simulink model "SPWM"  (R2019b)
settings: Solver=ode1  StartTime=0.0  StopTime=2  FixedStep=1e-5  RelTol=1e-3
InitFcn:
  | %T=0.0000071
  | T = (1e-5)/2
  | 
  | flux=0.2068
values from neighbouring files (symbols this model uses):
  B = 0.0136    [Pmsm.m]
  J = 0.0027    [Pmsm.m]
  Kiq = double(Kiq)    [Pmsm.m]
  Kiw = double(Kiw)    [Pmsm.m]
  Kpq = double(Kpq)    [Pmsm.m]
  Kpw = double(Kpw)    [Pmsm.m]
  Lambda_m = 0.2026    [Pmsm.m]
  Ld = 19.75e-3    (= 0.01975)    [Pmsm.m]
  Lq = 22.5e-3    (= 0.0225)    [Pmsm.m]
  P = 8    [Pmsm.m]
  Rs = 1.477    [Pmsm.m]
  Vdc = 220    [Pmsm.m]
libraries: modelsimlib x1
settings Model: Creator=samfi  LastModifiedBy=samfi

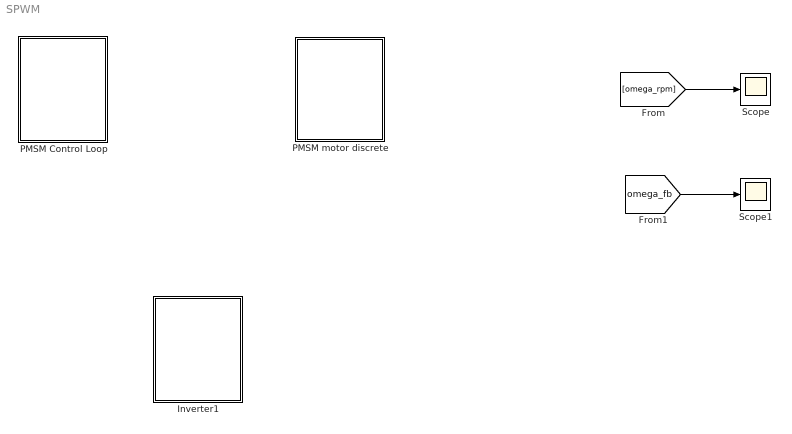
== system SPWM ==
  Inverter1 : Subsystem
  PMSM Control Loop : Subsystem
  PMSM motor discrete : Subsystem
  Scope : Scope
  Scope1 : Scope
  wires:
  [omega_rpm] -> Scope/1
  [omega_fb] -> Scope1/1

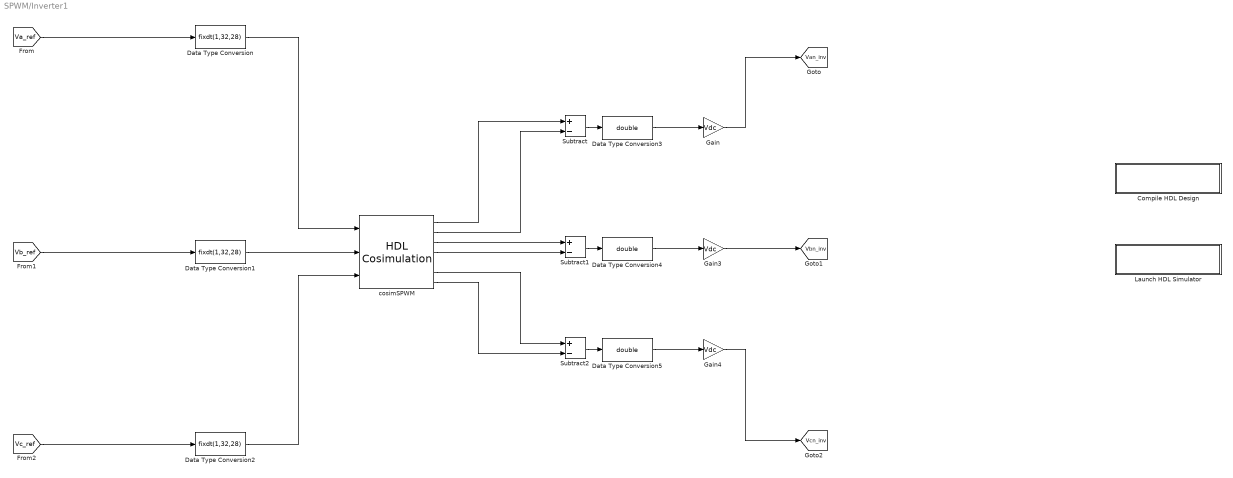
== system SPWM/Inverter1 ==
  Compile HDL Design : Subsystem
      settings: OpenFcn=eval('compile_hdl_design_cosimSPWM');
      mask Display: disp(['Double-Click to' char(10) 'compile HDL files'])
  Data Type Conversion : DataTypeConversion  OutDataTypeStr=fixdt(1,32,28)
  Data Type Conversion1 : DataTypeConversion  OutDataTypeStr=fixdt(1,32,28)
  Data Type Conversion2 : DataTypeConversion  OutDataTypeStr=fixdt(1,32,28)
  Data Type Conversion3 : DataTypeConversion  OutDataTypeStr=double
  Data Type Conversion4 : DataTypeConversion  OutDataTypeStr=double
  Data Type Conversion5 : DataTypeConversion  OutDataTypeStr=double
  Gain : Gain  Gain=Vdc
  Gain3 : Gain  Gain=Vdc
  Gain4 : Gain  Gain=Vdc
  Launch HDL Simulator : Subsystem
      settings: OpenFcn=eval('launch_hdl_simulator_cosimSPWM');
      mask Display: disp(['Double-Click to' char(10) 'launch HDL simulator'])
  Subtract : Sum  Inputs=+-
  Subtract1 : Sum  Inputs=+-
  Subtract2 : Sum  Inputs=+-
  cosimSPWM : modelsimlib/HDL Cosimulation  PortPaths=/cosimSPWM/x;/cosimSPWM/y;/cosimSPWM/z;/cosimSPWM/Sau;/cosimSPWM/Sal;/cosimSPWM/Sbu;/cosimSPWM/Sbl;/cosimSPWM/Scu;/cosimSPWM/Scl;/cosimSPWM/out;  PortModes=[1 1 1 2 2 2 2 2 2 2 ]  PortTimes=[-1,-1,-1,1e-4,1e-4,1e-4,1e-4,1e-4,1e-4,1e-4]  PortSigns=[-1,-1,-1,-1,-1,-1,-1,-1,-1,-1,]  PortFracLengths=[0,0,0,0,0,0,0,0,0,0]  CommLocal=on  CommSharedMemory=on  CommPortNumber=4449  CommShowInfo=on  ClockModes=[]  ClockTimes=[]  TclPreSimCommand=|  TclPostSimCommand=|  TimingMode=s  TimingScaleFactor=1  idxCellArray={'UNUSED_VAR'}  CosimBypass=Full Simulation  AllowDirectFeedthrough=on  ProductName=EDA Simulator Link MQ  RunAutoTimescale=on  HdlClocks=/cosimSPWM/clk 10 ns;  PreRunTime=10  PreRunTimeUnit=ns
      TclPreSimCommand=|
      | force /cosimSPWM/clk 0 0 ns, 1 5 ns -repeat 10 ns;
      | force /cosimSPWM/res 1 0 ns, 0 8 ns;
      TclPostSimCommand=|
      | noforce /cosimSPWM/clk;
      | noforce /cosimSPWM/res;
      | puts "done";
      settings: SourceProductName=HDL Verifier  SourceProductBaseCode=ES
  tag scope: Van_inv=global, Vbn_inv=global, Vcn_inv=global
  wires:
  [Vc_ref] -> Data Type Conversion2/1
  [Vb_ref] -> Data Type Conversion1/1
  [Va_ref] -> Data Type Conversion/1
  Data Type Conversion/1 -> cosimSPWM/1
  Data Type Conversion1/1 -> cosimSPWM/2
  Data Type Conversion2/1 -> cosimSPWM/3
  cosimSPWM/1 -> Subtract/1
  cosimSPWM/2 -> Subtract/2
  cosimSPWM/3 -> Subtract1/1
  cosimSPWM/4 -> Subtract1/2
  cosimSPWM/6 -> Subtract2/1
  cosimSPWM/7 -> Subtract2/2
  Subtract/1 -> Data Type Conversion3/1
  Subtract1/1 -> Data Type Conversion4/1
  Subtract2/1 -> Data Type Conversion5/1
  Gain4/1 -> [Vcn_inv]
  Gain3/1 -> [Vbn_inv]
  Gain/1 -> [Van_inv]
  Data Type Conversion3/1 -> Gain/1
  Data Type Conversion4/1 -> Gain3/1
  Data Type Conversion5/1 -> Gain4/1

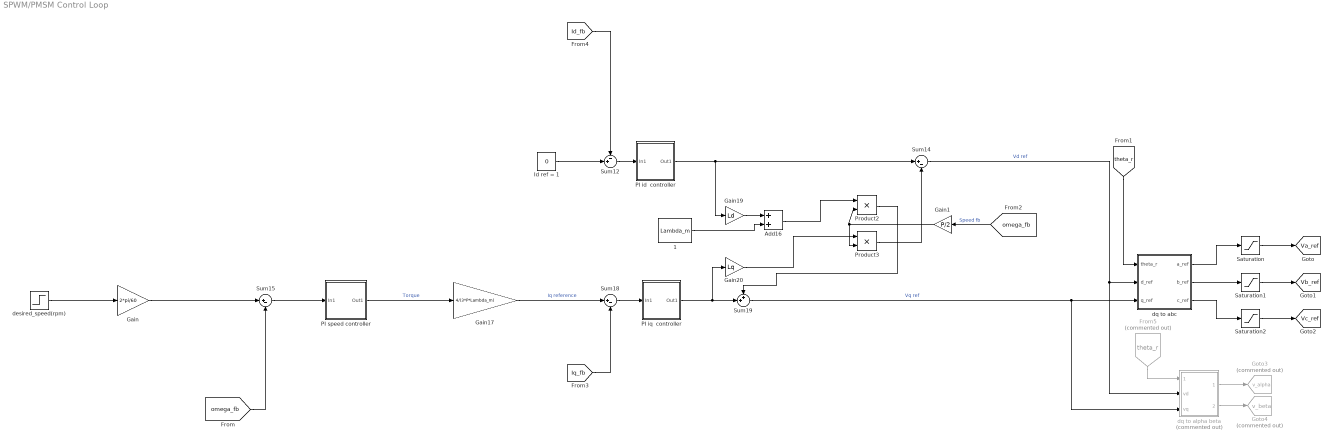
== system SPWM/PMSM Control Loop ==
  " 1" : Constant  Value=Lambda_m  SampleTime=1e-4
  Add16 : Sum
  From5 : From  Commented=on  GotoTag=theta_r  TagVisibility=global
  Gain : Gain  Gain=2*pi/60
  Gain1 : Gain  Gain=P/2
  Gain17 : Gain  Gain=4/(3*P*Lambda_m)
  Gain19 : Gain  Gain=Ld
  Gain20 : Gain  Gain=Lq
  Goto3 : Goto  Commented=on  GotoTag=v_alpha  TagVisibility=global
  Goto4 : Goto  Commented=on  GotoTag=v_beta  TagVisibility=global
  Id ref = 1 : Constant  Value=0  SampleTime=1e-4
  PI id  controller : Subsystem
  PI iq  controller : Subsystem
  PI speed controller : Subsystem
  Product2 : Product
  Product3 : Product
  Saturation : Saturate  UpperLimit=200  LowerLimit=-200
  Saturation1 : Saturate  UpperLimit=200  LowerLimit=-200
  Saturation2 : Saturate  UpperLimit=200  LowerLimit=-200
  Sum12 : Sum  Inputs=-+|
  Sum14 : Sum  Inputs=|+-
  Sum15 : Sum  Inputs=|+-
  Sum18 : Sum  Inputs=|+-
  Sum19 : Sum  Inputs=++|
  desired_speed(rpm) : Step  Time=0.25  After=400  SampleTime=1e-4
  dq to abc : Subsystem
  dq to alpha beta : Subsystem  Commented=on
  tag scope: Va_ref=global, Vb_ref=global, Vc_ref=global
  wires:
  Product2/1 -> Sum19/1
  Add16/1 -> Product2/1
  Gain20/1 -> Product3/1
  Product3/1 -> Sum14/2
  Id ref = 1/1 -> Sum12/2
  PI iq  controller/1(Out1) -> Gain20/1, Sum19/2
  PI id  controller/1(Out1) -> Gain19/1, Sum14/1
  Sum14/1 -> dq to alpha beta/2(vd), dq to abc/2(d_ref)  "Vd ref"
  Gain19/1 -> Add16/1
  Sum18/1 -> PI iq  controller/1(In1)
  " 1"/1 -> Add16/2
  Gain17/1 -> Sum18/1  "Iq reference"
  Sum19/1 -> dq to alpha beta/3(vq), dq to abc/3(q_ref)  "Vq ref"
  [omega_fb] -> Sum15/2
  [theta_r] -> dq to abc/1(theta_r)
  [Iq_fb] -> Sum18/2
  [Id_fb] -> Sum12/1
  Saturation/1 -> [Va_ref]
  Saturation1/1 -> [Vb_ref]
  Saturation2/1 -> [Vc_ref]
  dq to abc/3(c_ref) -> Saturation2/1
  dq to abc/1(a_ref) -> Saturation/1
  dq to abc/2(b_ref) -> Saturation1/1
  Gain/1 -> Sum15/1
  [omega_fb] -> Gain1/1  "Speed fb"
  Gain1/1 -> Product3/2, Product2/2
  Sum12/1 -> PI id  controller/1(In1)
  Sum15/1 -> PI speed controller/1(In1)
  PI speed controller/1(Out1) -> Gain17/1  "Torque"
  dq to alpha beta/1(valpha) -> Goto3/1
  dq to alpha beta/2(vbeta) -> Goto4/1
  From5/1 -> dq to alpha beta/1(theta_r)
  desired_speed(rpm)/1 -> Gain/1

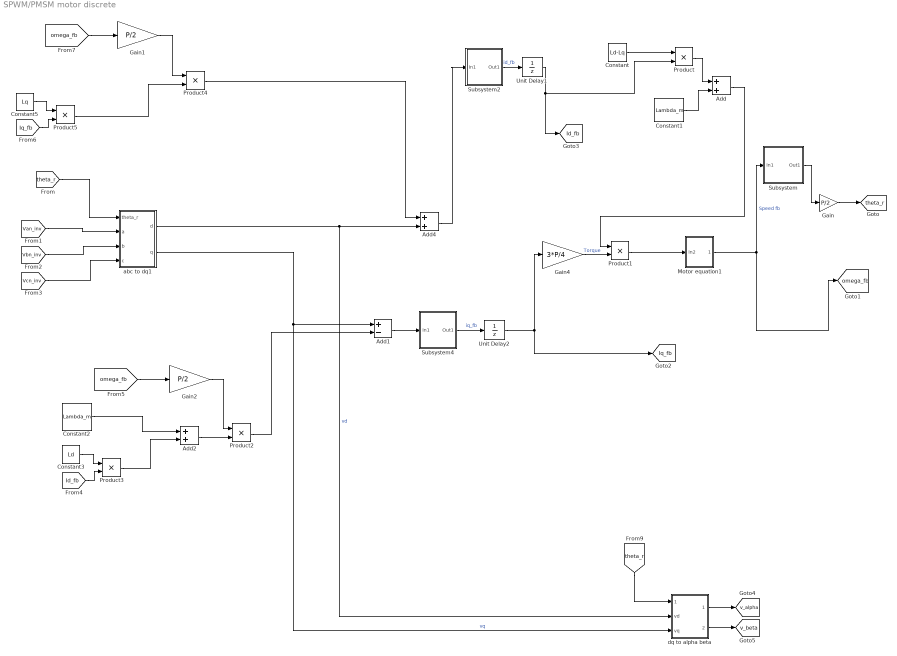
== system SPWM/PMSM motor discrete ==
  Add : Sum
  Add1 : Sum  Inputs=+-
  Add2 : Sum
  Add4 : Sum
  Constant : Constant  Value=Ld-Lq  SampleTime=1e-4
  Constant1 : Constant  Value=Lambda_m  SampleTime=1e-4
  Constant2 : Constant  Value=Lambda_m  SampleTime=1e-4
  Constant3 : Constant  Value=Ld  SampleTime=1e-4
  Constant5 : Constant  Value=Lq  SampleTime=1e-4
  Gain : Gain  Gain=P/2
  Gain1 : Gain  Gain=P/2
  Gain2 : Gain  Gain=P/2
  Gain4 : Gain  Gain=3*P/4
  Motor equation1 : Subsystem
  Product{,1..5} (6 alike) : Product
  Subsystem : Subsystem
  Subsystem2 : Subsystem
  Subsystem4 : Subsystem
  Unit Delay1 : UnitDelay  SampleTime=-1  HasFrameUpgradeWarning=on
  Unit Delay2 : UnitDelay  SampleTime=-1  HasFrameUpgradeWarning=on
  abc to dq1 : Subsystem
  dq to alpha beta : Subsystem
  tag scope: Id_fb=global, Iq_fb=global, omega_fb=global, theta_r=global, v_alpha=global, v_beta=global
  wires:
  Subsystem4/1(Out1) -> Unit Delay2/1  "iq_fb"
  [Vbn_inv] -> abc to dq1/3(b)
  Motor equation1/1(Out1) -> [omega_fb], Subsystem/1(In1)  "Speed fb"
  [Van_inv] -> abc to dq1/2(a)
  [Vcn_inv] -> abc to dq1/4(c)
  Subsystem2/1(Out1) -> Unit Delay1/1  "id_fb"
  Product1/1 -> Motor equation1/1(In2)
  Constant/1 -> Product/1
  Product/1 -> Add/1
  Constant1/1 -> Add/2
  Gain4/1 -> Product1/2  "Torque"
  Add/1 -> Product1/1
  Subsystem/1(Out1) -> Gain/1
  Gain/1 -> [theta_r]
  abc to dq1/2(q) -> dq to alpha beta/3(vq), Add1/1  "vq"
  Product2/1 -> Add1/2
  [omega_fb] -> Gain2/1
  Constant3/1 -> Product3/1
  [Id_fb] -> Product3/2
  Product3/1 -> Add2/2
  Constant2/1 -> Add2/1
  Add2/1 -> Product2/2
  [Iq_fb] -> Product5/2
  Product5/1 -> Product4/2
  Constant5/1 -> Product5/1
  abc to dq1/1(d) -> dq to alpha beta/2(vd), Add4/2  "vd"
  Product4/1 -> Add4/1
  [omega_fb] -> Gain1/1
  Gain1/1 -> Product4/1
  Gain2/1 -> Product2/1
  dq to alpha beta/1(valpha) -> [v_alpha]
  dq to alpha beta/2(vbeta) -> [v_beta]
  [theta_r] -> abc to dq1/1(theta_r)
  [theta_r] -> dq to alpha beta/1(theta_r)
  Add4/1 -> Subsystem2/1(In1)
  Add1/1 -> Subsystem4/1(In1)
  Unit Delay1/1 -> [Id_fb], Product/2
  Unit Delay2/1 -> Gain4/1, [Iq_fb]

== system SPWM/Inverter1/Compile HDL Design ==

== system SPWM/Inverter1/Launch HDL Simulator ==

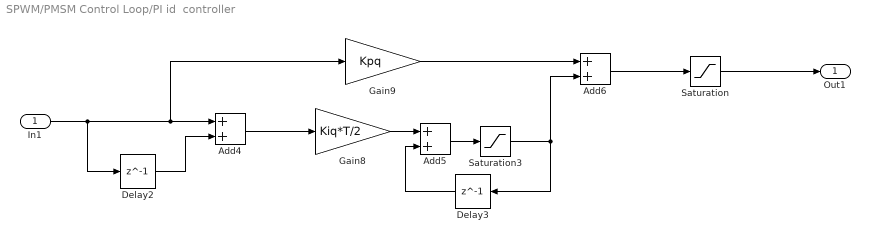
== system SPWM/PMSM Control Loop/PI id  controller ==
  In1 : Inport
  Add4 : Sum
  Add5 : Sum
  Add6 : Sum
  Delay2 : Delay  DelayLength=1
  Delay3 : Delay  DelayLength=1
  Gain8 : Gain  Gain=Kiq*T/2
  Gain9 : Gain  Gain=Kpq
  Saturation : Saturate  UpperLimit=220  LowerLimit=-220
  Saturation3 : Saturate  UpperLimit=200  LowerLimit=-200
  Out1 : Outport
  wires:
  Gain8/1 -> Add5/1
  Delay2/1 -> Add4/2
  Add5/1 -> Saturation3/1
  Add4/1 -> Gain8/1
  Saturation3/1 -> Delay3/1, Add6/2
  In1/1 -> Add4/1, Gain9/1, Delay2/1
  Gain9/1 -> Add6/1
  Delay3/1 -> Add5/2
  Add6/1 -> Saturation/1
  Saturation/1 -> Out1/1

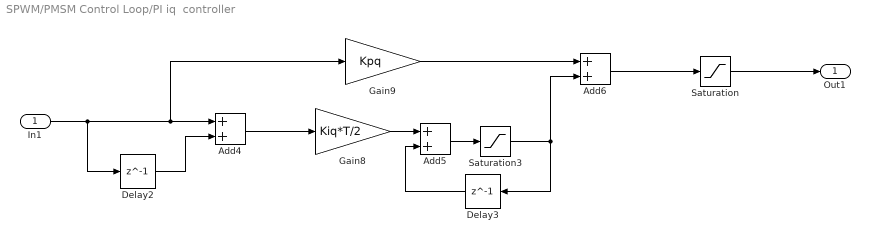
== system SPWM/PMSM Control Loop/PI iq  controller ==
  In1 : Inport
  Add4 : Sum
  Add5 : Sum
  Add6 : Sum
  Delay2 : Delay  DelayLength=1
  Delay3 : Delay  DelayLength=1
  Gain8 : Gain  Gain=Kiq*T/2
  Gain9 : Gain  Gain=Kpq
  Saturation : Saturate  UpperLimit=220  LowerLimit=-220
  Saturation3 : Saturate  UpperLimit=200  LowerLimit=-200
  Out1 : Outport
  wires:
  Delay3/1 -> Add5/2
  Gain9/1 -> Add6/1
  In1/1 -> Delay2/1, Gain9/1, Add4/1
  Saturation3/1 -> Add6/2, Delay3/1
  Add4/1 -> Gain8/1
  Add5/1 -> Saturation3/1
  Delay2/1 -> Add4/2
  Gain8/1 -> Add5/1
  Add6/1 -> Saturation/1
  Saturation/1 -> Out1/1

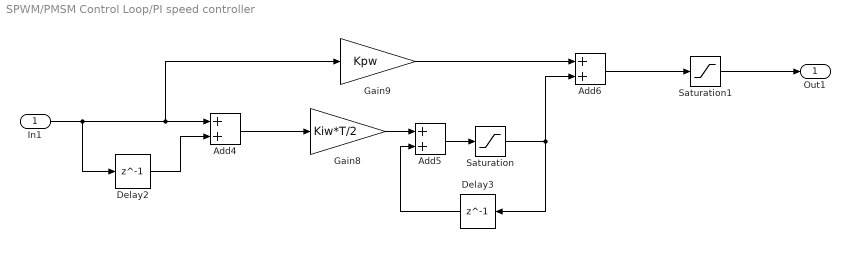
== system SPWM/PMSM Control Loop/PI speed controller ==
  In1 : Inport
  Add4 : Sum
  Add5 : Sum
  Add6 : Sum
  Delay2 : Delay  DelayLength=1
  Delay3 : Delay  DelayLength=1
  Gain8 : Gain  Gain=Kiw*T/2
  Gain9 : Gain  Gain=Kpw
  Saturation : Saturate  UpperLimit=10  LowerLimit=-10
  Saturation1 : Saturate  UpperLimit=10  LowerLimit=-10
  Out1 : Outport
  wires:
  Gain9/1 -> Add6/1
  Delay2/1 -> Add4/2
  Gain8/1 -> Add5/1
  Add5/1 -> Saturation/1
  In1/1 -> Delay2/1, Gain9/1, Add4/1
  Saturation/1 -> Add6/2, Delay3/1
  Add4/1 -> Gain8/1
  Delay3/1 -> Add5/2
  Add6/1 -> Saturation1/1
  Saturation1/1 -> Out1/1

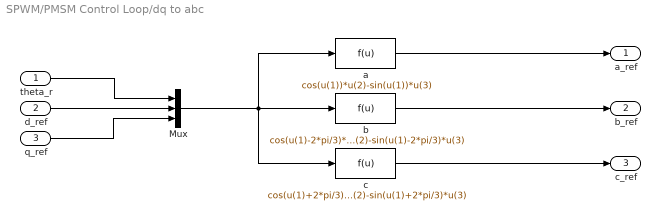
== system SPWM/PMSM Control Loop/dq to abc ==
  theta_r : Inport
  d_ref : Inport  Port=2
  q_ref : Inport  Port=3
  Mux : Mux  Inputs=3
  a : Fcn  Expr=cos(u(1))*u(2)-sin(u(1))*u(3)
  b : Fcn  Expr=cos(u(1)-2*pi/3)*u(2)-sin(u(1)-2*pi/3)*u(3)
  c : Fcn  Expr=cos(u(1)+2*pi/3)*u(2)-sin(u(1)+2*pi/3)*u(3)
  a_ref : Outport
  b_ref : Outport  Port=2
  c_ref : Outport  Port=3
  wires:
  d_ref/1 -> Mux/2
  Mux/1 -> c/1, b/1, a/1
  c/1 -> c_ref/1
  theta_r/1 -> Mux/1
  b/1 -> b_ref/1
  a/1 -> a_ref/1
  q_ref/1 -> Mux/3

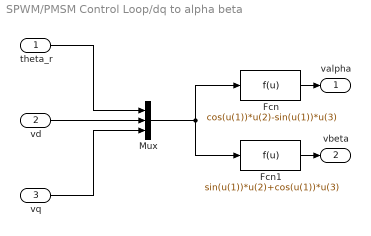
== system SPWM/PMSM Control Loop/dq to alpha beta ==
  theta_r : Inport
  vd : Inport  Port=2
  vq : Inport  Port=3
  Fcn : Fcn  Expr=cos(u(1))*u(2)-sin(u(1))*u(3)
  Fcn1 : Fcn  Expr=sin(u(1))*u(2)+cos(u(1))*u(3)
  Mux : Mux  Inputs=3
  valpha : Outport
  vbeta : Outport  Port=2
  wires:
  Mux/1 -> Fcn/1, Fcn1/1
  vq/1 -> Mux/3
  theta_r/1 -> Mux/1
  Fcn1/1 -> vbeta/1
  vd/1 -> Mux/2
  Fcn/1 -> valpha/1

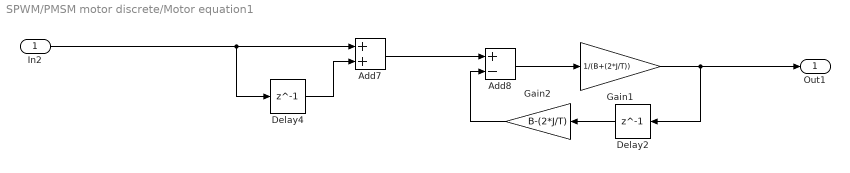
== system SPWM/PMSM motor discrete/Motor equation1 ==
  In2 : Inport
  Add7 : Sum
  Add8 : Sum  Inputs=+-
  Delay2 : Delay  DelayLength=1
  Delay4 : Delay  DelayLength=1
  Gain1 : Gain  Gain=1/(B+(2*J/T))
  Gain2 : Gain  Gain=B-(2*J/T)
  Out1 : Outport
  wires:
  Add7/1 -> Add8/1
  Gain1/1 -> Out1/1, Delay2/1
  Delay2/1 -> Gain2/1
  Add8/1 -> Gain1/1
  Gain2/1 -> Add8/2
  In2/1 -> Delay4/1, Add7/1
  Delay4/1 -> Add7/2

== system SPWM/PMSM motor discrete/Subsystem ==
  In1 : Inport
  Add1 : Sum
  Add2 : Sum
  Delay1 : Delay  DelayLength=1
  Delay4 : Delay  DelayLength=1
  Gain : Gain  Gain=T/2
  Out1 : Outport
  wires:
  In1/1 -> Delay4/1, Add1/1
  Delay1/1 -> Add2/2
  Add2/1 -> Out1/1, Delay1/1
  Delay4/1 -> Add1/2
  Add1/1 -> Gain/1
  Gain/1 -> Add2/1

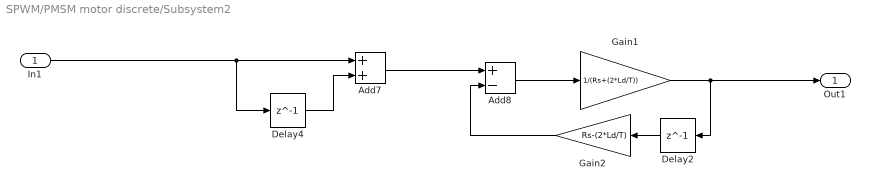
== system SPWM/PMSM motor discrete/Subsystem2 ==
  In1 : Inport
  Add7 : Sum
  Add8 : Sum  Inputs=+-
  Delay2 : Delay  DelayLength=1
  Delay4 : Delay  DelayLength=1
  Gain1 : Gain  Gain=1/(Rs+(2*Ld/T))
  Gain2 : Gain  Gain=Rs-(2*Ld/T)
  Out1 : Outport
  wires:
  Add8/1 -> Gain1/1
  In1/1 -> Add7/1, Delay4/1
  Gain2/1 -> Add8/2
  Delay2/1 -> Gain2/1
  Delay4/1 -> Add7/2
  Add7/1 -> Add8/1
  Gain1/1 -> Out1/1, Delay2/1

== system SPWM/PMSM motor discrete/Subsystem4 ==
  In1 : Inport
  Add7 : Sum
  Add8 : Sum  Inputs=+-
  Delay2 : Delay  DelayLength=1
  Delay4 : Delay  DelayLength=1
  Gain1 : Gain  Gain=1/(Rs+(2*Lq/T))
  Gain2 : Gain  Gain=Rs-(2*Lq/T)
  Out1 : Outport
  wires:
  Add8/1 -> Gain1/1
  Gain1/1 -> Delay2/1, Out1/1
  Add7/1 -> Add8/1
  Delay4/1 -> Add7/2
  Delay2/1 -> Gain2/1
  Gain2/1 -> Add8/2
  In1/1 -> Delay4/1, Add7/1

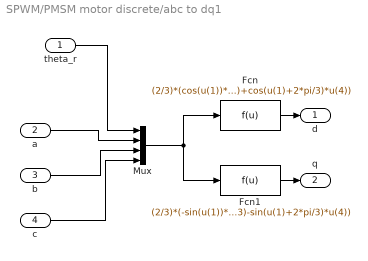
== system SPWM/PMSM motor discrete/abc to dq1 ==
  theta_r : Inport
  a : Inport  Port=2
  b : Inport  Port=3
  c : Inport  Port=4
  Fcn : Fcn  Expr=(2/3)*(cos(u(1))*u(2)+cos(u(1)-2*pi/3)*u(3)+cos(u(1)+2*pi/3)*u(4))
  Fcn1 : Fcn  Expr=(2/3)*(-sin(u(1))*u(2)-sin(u(1)-2*pi/3)*u(3)-sin(u(1)+2*pi/3)*u(4))
  Mux : Mux
  d : Outport
  q : Outport  Port=2
  wires:
  a/1 -> Mux/2
  c/1 -> Mux/4
  theta_r/1 -> Mux/1
  Mux/1 -> Fcn/1, Fcn1/1
  b/1 -> Mux/3
  Fcn/1 -> d/1
  Fcn1/1 -> q/1

== system SPWM/PMSM motor discrete/dq to alpha beta ==
  theta_r : Inport
  vd : Inport  Port=2
  vq : Inport  Port=3
  Fcn : Fcn  Expr=cos(u(1))*u(2)-sin(u(1))*u(3)
  Fcn1 : Fcn  Expr=sin(u(1))*u(2)+cos(u(1))*u(3)
  Mux : Mux  Inputs=3
  valpha : Outport
  vbeta : Outport  Port=2
  wires:
  Mux/1 -> Fcn/1, Fcn1/1
  vq/1 -> Mux/3
  theta_r/1 -> Mux/1
  Fcn1/1 -> vbeta/1
  vd/1 -> Mux/2
  Fcn/1 -> valpha/1
